simulink model "planmodel2023"  (R2023b)
settings: Solver=ode4  StartTime=0.0  StopTime=200  FixedStep=0.001  RelTol=1e-3
values from neighbouring files (symbols this model uses):
  a0 = 340.294    [plan.m]    (also in plan.mat)
  b_ref = 2.0    (= 2)    [plan.m]    (also in plan.mat)
  c_gear = [0.8e4, 1.4e4, 1.4e4]    [plan.m]    (also in plan.mat = [8000 14000 14000])
  c_lat = [1.4e4, 2.2e4, 2.2e4]    [plan.m]    (also in plan.mat = [14000 22000 22000])
  c_ref = 0.9    [plan.m]    (also in plan.mat)
  c_roll = [0.020, 0.018, 0.018]    [plan.m]    (also in plan.mat = [0.02 0.018 0.018])
  CD0 = 0.045    [plan.m]    (also in plan.mat)
  CL0 = 0.083    [plan.m]    (also in plan.mat)
  CLa = 2.50    (= 2.5)    [plan.m]    (also in plan.mat = 3.8)
  Clb = -0.08    [plan.m]    (also in plan.mat)
  Clda = 0.20    (= 0.2)    [plan.m]    (also in plan.mat = -0.2)
  CLde = 0.25    [plan.m]    (also in plan.mat = 0.28)
  Clp = -0.70    (= -0.7)    [plan.m]    (also in plan.mat)
  CLq = 3.00    (= 3)    [plan.m]    (also in plan.mat = 4.5)
  Clr = 0    [plan.m]    (also in plan.mat = 0.08)
  Cm0 = 0.112    [plan.m]    (also in plan.mat = 0.06)
  Cma = -0.8    [plan.m]    (also in plan.mat)
  Cmde = 0.90    (= 0.9)    [plan.m]    (also in plan.mat = -0.9)
  Cmq = -18.0    (= -18)    [plan.m]    (also in plan.mat)
  Cnb = -0.25    [plan.m]    (also in plan.mat = 0.25)
  Cndr = 0.15    [plan.m]    (also in plan.mat = -0.15)
  Cnp = 0    [plan.m]    (also in plan.mat = -0.04)
  Cnr = -0.45    [plan.m]    (also in plan.mat)
  CSb = -0.8    [plan.m]    (also in plan.mat = -0.7)
  CSdr = 0.18    [plan.m]    (also in plan.mat)
  CSr = 0.15    [plan.m]    (also in plan.mat = 0.12)
  D0 = 800    [plan.m]    (also in plan.mat)
  da_max = 25    [plan.m]    (also in plan.mat)
  da_min = -da_max    (= -25)    [plan.m]    (also in plan.mat)
  de_max = 25    [plan.m]    (also in plan.mat)
  de_min = -de_max    (= -25)    [plan.m]    (also in plan.mat)
  DH = pi / 180    (= 0.0174532925199)    [plan.m]    (also in plan.mat)
  dr_max = 25    [plan.m]    (also in plan.mat)
  dr_min = -dr_max    (= -25)    [plan.m]    (also in plan.mat)
  g = 9.80665    [plan.m]    (also in plan.mat)
  gamma0 = 0.0    (= 0)    [plan.m]
  ground_y = 0.0    (= 0)    [plan.m]
  HD = 180 / pi    (= 57.2957795131)    [plan.m]    (also in plan.mat)
  Ixx = 120.0    (= 120)    [plan.m]    (also in plan.mat)
  Iyy = 480.0    (= 480)    [plan.m]    (also in plan.mat)
  Izz = 520.0    (= 520)    [plan.m]    (also in plan.mat)
  K = 0.080    (= 0.08)    [plan.m]    (also in plan.mat = 0.12)
  K_alpha = 7.67884615385    [plan.mat]
  k_gear = [1.0e5, 3.0e5, 3.0e5]    [plan.m]    (also in plan.mat = [100000 300000 300000])
  k_theta0 = 0.0    (= 0)    [plan.m]
  Kb_to_wy = 10.6510416667    [plan.mat]
  Kn_pitch = 0.117046638908    [plan.mat]
  Kn_to_beta = 0.461367696223    [plan.mat]
  Kw_pitch = -0.524061476442    [plan.mat]
  Kw_to_dr = -1.30612244898    [plan.mat]
  m = 600.0    (= 600)    [plan.m]    (also in plan.mat)
  mu_brake = [0.0, 0.55, 0.55]    [plan.m]    (also in plan.mat = [0 0.55 0.55])
  omigax0 = 0    [plan.m]
  omigay0 = 0    [plan.m]
  omigaz0 = 0    [plan.m]
  psi0 = 0.3/57.3    (= 0.00523560209424)    [plan.m]    (also in plan.mat = 0)
  r_left_b = r_gear_b(:,2)    [plan.m]    (also in plan.mat = [-0.333333333333 -0.8 0.65])
  r_nose_b = r_gear_b(:,1)    [plan.m]    (also in plan.mat = [2 0 0.65])
  r_right_b = r_gear_b(:,3)    [plan.m]    (also in plan.mat = [-0.333333333333 0.8 0.65])
  rho0 = 1.225    [plan.m]    (also in plan.mat)
  S_ref = 1.2    [plan.m]    (also in plan.mat)
  v_eps = 0.20    (= 0.2)    [plan.m]    (also in plan.mat)
  V_min = 1    [plan.m]    (also in plan.mat = 3)
  V_test = 200    [plan.mat]
  Vx0_b = 0.0    (= 0)    [plan.m]
  Vy0_b = 0.0    (= 0)    [plan.m]
  Vz0_b = 0.0    (= 0)    [plan.m]
  wheel_radius = 0.18    [plan.m]    (also in plan.mat)
  WOW_on = 0.000    (= 0)    [plan.m]    (also in plan.mat)
  Xg0 = 0.0    (= 0)    [plan.m]    (also in plan.mat)
  Yg0 = ground_y + wheel_radius - r_gear_b(2,1) - static_deflection    [plan.m]    (also in plan.mat = 0)
  Zg0 = 1.0    (= 1)    [plan.m]    (also in plan.mat = -0.8215943)
libraries: matrix_library x18, slpidlib x1
(part 2 of 3)

== system planmodel2023/control/航向通道控制器/偏航通道 ==
  nzc : Inport
  nz : Inport  Port=2
  wy : Inport  Port=3
  Constant1 : Constant
  Constant3 : Constant  Value=0
  Div : Product  Inputs=/*
  Gain : Gain  Gain=-Kn_to_beta
  Gain1 : Gain  Gain=Kb_to_wy
  Gain2 : Gain  Gain=Kw_to_dr
  Gain4 : Gain  Gain=HD
  Integrator : Integrator  ExternalReset=either
  Pk : Product
  Pn : Product
  Sat : Saturate  UpperLimit=10  LowerLimit=0.25
  Saturation1 : Saturate  UpperLimit=0.2*57.3  LowerLimit=-0.2*57.3
  Scope : Scope  NumInputPorts=2
  Scope1 : Scope
  Scope12 : Scope
  Scope2 : Scope  NumInputPorts=2
  Sqr : Math  Operator=square
  Sum : Sum  Inputs=|+-
  Sum1 : Sum  Inputs=|+-
  Sum2 : Sum  Inputs=|+-
  Switch2 : Switch  Threshold=40  SaturateOnIntegerOverflow=off  InputSameDT=off
  VRef : Constant  Value=V_test
  伪攻角回路 : Subsystem
  delta_r : Outport
  wires:
  nz/1 -> Sum/2, Scope/2
  nzc/1 -> Scope/1, Sum/1
  Constant1/1 -> Switch2/1
  Constant3/1 -> Switch2/3
  [Vg] -> Div/2, Switch2/2
  Gain4/1 -> Scope12/1
  [psi_eular] -> Gain4/1
  wy/1 -> Scope2/2, Sum2/2, 伪攻角回路/1(wy)
  伪攻角回路/1(beta_c) -> Sum1/2
  Sum1/1 -> Gain1/1
  Gain1/1 -> Scope2/1, Sum2/1
  Sum2/1 -> Gain2/1
  Sum/1 -> Gain/1
  Integrator/1 -> Saturation1/1
  Saturation1/1 -> Sum1/1
  Switch2/1 -> Integrator/2
  VRef/1 -> Div/1
  Div/1 -> Sqr/1
  Sqr/1 -> Sat/1
  Sat/1 -> Pn/2, Pk/2
  Gain2/1 -> Pk/1
  Pk/1 -> delta_r/1, Scope1/1
  Gain/1 -> Pn/1
  Pn/1 -> Integrator/1

== system planmodel2023/control/航向通道控制器/地面转向控制 ==
  Z_cmd : Inport
  Gain : Gain  Gain=0.8
  Gain4 : Gain  Gain=HD
  K_z : Constant  Value=0.04
  Product : Product
  Saturation1 : Saturate  UpperLimit=5  LowerLimit=-5
  Scope : Scope  NumInputPorts=2
  Scope12 : Scope
  Scope25 : Scope
  Sum : Sum  Inputs=|+-
  Sum1 : Sum  Inputs=|++
  Transfer Fcn : TransferFcn  Denominator=[0.1 1]
  delta_s(H) : Outport
  wires:
  Z_cmd/1 -> Scope/1, Sum/1
  [Z_positon] -> Scope/2, Sum/2
  K_z/1 -> Product/1
  [delta_s] -> Scope25/1
  [psi_eular] -> Gain/1
  Gain4/1 -> Scope12/1
  [psi_eular] -> Gain4/1
  Gain/1 -> Sum1/2
  Sum/1 -> Saturation1/1
  Product/1 -> Sum1/1
  Saturation1/1 -> Product/2
  Sum1/1 -> Transfer Fcn/1
  Transfer Fcn/1 -> delta_s(H)/1

== system planmodel2023/control/航向通道控制器1/偏航通道 ==
  nzc : Inport
  nz : Inport  Port=2
  wy : Inport  Port=3
  Constant1 : Constant
  Constant3 : Constant  Value=0
  Gain : Gain  Gain=-Kn_to_beta
  Gain1 : Gain  Gain=Kb_to_wy
  Gain2 : Gain  Gain=Kw_to_dr
  Gain4 : Gain  Gain=HD
  Integrator : Integrator  ExternalReset=either
  Saturation1 : Saturate  UpperLimit=0.2*57.3  LowerLimit=-0.2*57.3
  Scope : Scope  NumInputPorts=2
  Scope1 : Scope
  Scope12 : Scope
  Scope2 : Scope  NumInputPorts=2
  Sum : Sum  Inputs=|+-
  Sum1 : Sum  Inputs=|+-
  Sum2 : Sum  Inputs=|+-
  Switch2 : Switch  Threshold=40  SaturateOnIntegerOverflow=off  InputSameDT=off
  伪攻角回路 : Subsystem
  delta_r : Outport
  wires:
  nz/1 -> Scope/2, Sum/2
  nzc/1 -> Scope/1, Sum/1
  Constant1/1 -> Switch2/1
  Constant3/1 -> Switch2/3
  [Vg] -> Switch2/2
  Gain4/1 -> Scope12/1
  [psi_eular] -> Gain4/1
  wy/1 -> Scope2/2, Sum2/2, 伪攻角回路/1(wy)
  伪攻角回路/1(beta_c) -> Sum1/2
  Sum1/1 -> Gain1/1
  Gain1/1 -> Scope2/1, Sum2/1
  Sum2/1 -> Gain2/1
  Gain2/1 -> Scope1/1, delta_r/1
  Gain/1 -> Integrator/1
  Sum/1 -> Gain/1
  Integrator/1 -> Saturation1/1
  Saturation1/1 -> Sum1/1
  Switch2/1 -> Integrator/2

== system planmodel2023/control/航向通道控制器1/地面转向控制 ==
  Z_cmd : Inport
  Gain : Gain  Gain=0.8
  Gain4 : Gain  Gain=HD
  K_z : Constant  Value=0.04
  Product : Product
  Saturation1 : Saturate  UpperLimit=5  LowerLimit=-5
  Scope : Scope  NumInputPorts=2
  Scope12 : Scope
  Scope25 : Scope
  Sum : Sum  Inputs=|+-
  Sum1 : Sum  Inputs=|++
  delta_s(H) : Outport
  wires:
  Z_cmd/1 -> Scope/1, Sum/1
  [Z_positon] -> Scope/2, Sum/2
  K_z/1 -> Product/1
  [delta_s] -> Scope25/1
  [psi_eular] -> Gain/1
  Gain4/1 -> Scope12/1
  [psi_eular] -> Gain4/1
  Gain/1 -> Sum1/2
  Sum/1 -> Saturation1/1
  Product/1 -> Sum1/1
  Saturation1/1 -> Product/2
  Sum1/1 -> delta_s(H)/1

== system planmodel2023/6DOF-MODEL/AERO-PARAMETER/无量纲化角速率/Subsystem ==
  wy1 : Inport
  Va : Inport  Port=2
  Constant4 : Constant  Value=b_ref
  Divide : Product  Inputs=*/
  Gain : Gain  Gain=2
  Product : Product
  r_hat : Outport
  wires:
  Va/1 -> Gain/1
  wy1/1 -> Product/1
  Constant4/1 -> Product/2
  Product/1 -> Divide/1
  Divide/1 -> r_hat/1
  Gain/1 -> Divide/2

== system planmodel2023/6DOF-MODEL/AERO-PARAMETER/无量纲化角速率/Subsystem1 ==
  wz1 : Inport
  Va : Inport  Port=2
  Constant4 : Constant  Value=c_ref
  Divide : Product  Inputs=*/
  Gain : Gain  Gain=2
  Product : Product
  Scope : Scope
  q_hat : Outport
  wires:
  Va/1 -> Gain/1
  wz1/1 -> Scope/1, Product/1
  Constant4/1 -> Product/2
  Product/1 -> Divide/1
  Divide/1 -> q_hat/1
  Gain/1 -> Divide/2

== system planmodel2023/6DOF-MODEL/AERO-PARAMETER/无量纲化角速率/Subsystem2 ==
  wx1 : Inport
  Va : Inport  Port=2
  Constant4 : Constant  Value=b_ref
  Divide : Product  Inputs=*/
  Gain : Gain  Gain=2
  Product : Product
  p_hat : Outport
  wires:
  Va/1 -> Gain/1
  wx1/1 -> Product/1
  Constant4/1 -> Product/2
  Product/1 -> Divide/1
  Divide/1 -> p_hat/1
  Gain/1 -> Divide/2

== system planmodel2023/6DOF-MODEL/动力学/v在体系下的分量/Subsystem ==
  Fx/m : Inport
  wy1 : Inport  Port=2
  wz1 : Inport  Port=3
  vz : Inport  Port=4
  vy : Inport  Port=5
  Product1 : Product
  Product4 : Product
  Subtract1 : Sum  Inputs=+-
  Subtract3 : Sum  Inputs=+-
  vx_dot : Outport
  wires:
  Fx/m/1 -> Subtract3/1
  Subtract3/1 -> vx_dot/1
  Subtract1/1 -> Subtract3/2
  vy/1 -> Product4/2
  wz1/1 -> Product4/1
  Product4/1 -> Subtract1/2
  wy1/1 -> Product1/1
  vz/1 -> Product1/2
  Product1/1 -> Subtract1/1

== system planmodel2023/6DOF-MODEL/动力学/v在体系下的分量/Subsystem1 ==
  Fy/m : Inport
  wx1 : Inport  Port=2
  wz1 : Inport  Port=3
  vx : Inport  Port=4
  vz : Inport  Port=5
  Product1 : Product
  Product4 : Product
  Subtract2 : Sum  Inputs=+-
  Subtract3 : Sum  Inputs=+-
  vy_dot : Outport
  wires:
  Fy/m/1 -> Subtract3/1
  Subtract3/1 -> vy_dot/1
  vx/1 -> Product4/1
  wz1/1 -> Product4/2
  wx1/1 -> Product1/1
  vz/1 -> Product1/2
  Product4/1 -> Subtract2/1
  Product1/1 -> Subtract2/2
  Subtract2/1 -> Subtract3/2

== system planmodel2023/6DOF-MODEL/动力学/v在体系下的分量/Subsystem2 ==
  Fz/m : Inport
  wx1 : Inport  Port=2
  wy1 : Inport  Port=3
  vx : Inport  Port=4
  vy : Inport  Port=5
  Product1 : Product
  Product2 : Product
  Subtract2 : Sum  Inputs=+-
  Subtract3 : Sum  Inputs=+-
  vz_dot : Outport
  wires:
  Fz/m/1 -> Subtract3/1
  Subtract3/1 -> vz_dot/1
  Subtract2/1 -> Subtract3/2
  Product1/1 -> Subtract2/1
  wx1/1 -> Product1/1
  vy/1 -> Product1/2
  wy1/1 -> Product2/1
  vx/1 -> Product2/2
  Product2/1 -> Subtract2/2

== system planmodel2023/6DOF-MODEL/动力学/体系旋转角速度/Subsystem ==
  MX : Inport
  wz1 : Inport  Port=2
  wy1 : Inport  Port=3
  Constant : Constant  Value=Ixx
  Constant1 : Constant  Value=Izz
  Constant2 : Constant  Value=Iyy
  Divide : Product  Inputs=*/
  Integrator : Integrator  InitialCondition=omigax0
  Product : Product
  Product1 : Product
  Subtract : Sum  Inputs=+-
  Sum : Sum  Inputs=|+-
  wx1 : Outport
  wires:
  MX/1 -> Sum/1
  Sum/1 -> Divide/1
  Constant/1 -> Divide/2
  Subtract/1 -> Product/1
  wz1/1 -> Product1/1
  wy1/1 -> Product1/2
  Product1/1 -> Product/2
  Constant1/1 -> Subtract/1
  Constant2/1 -> Subtract/2
  Product/1 -> Sum/2
  Divide/1 -> Integrator/1
  Integrator/1 -> wx1/1

== system planmodel2023/6DOF-MODEL/动力学/体系旋转角速度/Subsystem1 ==
  MY : Inport
  wx1 : Inport  Port=2
  wz1 : Inport  Port=3
  Constant : Constant  Value=Iyy
  Constant1 : Constant  Value=Ixx
  Constant2 : Constant  Value=Izz
  Divide : Product  Inputs=*/
  Integrator : Integrator  InitialCondition=omigay0
  Product : Product
  Product1 : Product
  Subtract : Sum  Inputs=+-
  Sum : Sum  Inputs=|+-
  wy1 : Outport
  wires:
  MY/1 -> Sum/1
  Sum/1 -> Divide/1
  Constant/1 -> Divide/2
  Subtract/1 -> Product/1
  wx1/1 -> Product1/1
  wz1/1 -> Product1/2
  Product1/1 -> Product/2
  Constant1/1 -> Subtract/1
  Constant2/1 -> Subtract/2
  Product/1 -> Sum/2
  Divide/1 -> Integrator/1
  Integrator/1 -> wy1/1

== system planmodel2023/6DOF-MODEL/动力学/体系旋转角速度/Subsystem2 ==
  MZ : Inport
  wx1 : Inport  Port=2
  wy1 : Inport  Port=3
  Constant : Constant  Value=Izz
  Constant1 : Constant  Value=Iyy
  Constant2 : Constant  Value=Ixx
  Divide : Product  Inputs=*/
  Integrator : Integrator  InitialCondition=omigaz0
  Product : Product
  Product1 : Product
  Subtract : Sum  Inputs=+-
  Sum : Sum  Inputs=|+-
  wz1 : Outport
  wires:
  MZ/1 -> Sum/1
  Sum/1 -> Divide/1
  Constant/1 -> Divide/2
  Subtract/1 -> Product/1
  wx1/1 -> Product1/1
  wy1/1 -> Product1/2
  Product1/1 -> Product/2
  Constant1/1 -> Subtract/1
  Constant2/1 -> Subtract/2
  Product/1 -> Sum/2
  Divide/1 -> Integrator/1
  Integrator/1 -> wz1/1

== system planmodel2023/6DOF-MODEL/动力学/姿态角/Subsystem ==
  wx1 : Inport
  wy1 : Inport  Port=2
  wz1 : Inport  Port=3
  Integrator : Integrator  InitialCondition=gamma0
  Product : Product
  Product1 : Product
  Product2 : Product
  Subtract : Sum  Inputs=+-
  Sum : Sum  Inputs=|+-
  Trigonometric Function1 : Trigonometry  Operator=cos
  Trigonometric Function2 : Trigonometry
  Trigonometric Function8 : Trigonometry  Operator=tan
  gamma(eular) : Outport
  wires:
  wx1/1 -> Sum/1
  [gamma_eular] -> Trigonometric Function2/1, Trigonometric Function1/1
  Trigonometric Function1/1 -> Product/2
  wy1/1 -> Product/1
  Trigonometric Function2/1 -> Product1/1
  wz1/1 -> Product1/2
  Product/1 -> Subtract/1
  Product1/1 -> Subtract/2
  Subtract/1 -> Product2/2
  [theta_eular] -> Trigonometric Function8/1
  Trigonometric Function8/1 -> Product2/1
  Sum/1 -> Integrator/1
  Integrator/1 -> gamma(eular)/1
  Product2/1 -> Sum/2

== system planmodel2023/6DOF-MODEL/动力学/姿态角/Subsystem1 ==
  wy1 : Inport
  wz1 : Inport  Port=2
  Integrator : Integrator  InitialCondition=k_theta0
  Product : Product
  Product1 : Product
  Subtract : Sum
  Trigonometric Function1 : Trigonometry
  Trigonometric Function2 : Trigonometry  Operator=cos
  theta(eular) : Outport
  wires:
  [gamma_eular] -> Trigonometric Function2/1, Trigonometric Function1/1
  Trigonometric Function1/1 -> Product/2
  wy1/1 -> Product/1
  Trigonometric Function2/1 -> Product1/1
  wz1/1 -> Product1/2
  Product/1 -> Subtract/1
  Product1/1 -> Subtract/2
  Subtract/1 -> Integrator/1
  Integrator/1 -> theta(eular)/1

== system planmodel2023/6DOF-MODEL/动力学/姿态角/Subsystem2 ==
  wy1 : Inport
  wz1 : Inport  Port=2
  Divide : Product  Inputs=*/
  Integrator : Integrator  InitialCondition=psi0
  Product : Product
  Product1 : Product
  Subtract : Sum  Inputs=+-
  Trigonometric Function1 : Trigonometry  Operator=cos
  Trigonometric Function2 : Trigonometry
  Trigonometric Function8 : Trigonometry  Operator=cos
  psi(eular) : Outport
  wires:
  [gamma_eular] -> Trigonometric Function2/1, Trigonometric Function1/1
  Trigonometric Function1/1 -> Product/2
  wy1/1 -> Product/1
  Trigonometric Function2/1 -> Product1/1
  wz1/1 -> Product1/2
  Product/1 -> Subtract/1
  Product1/1 -> Subtract/2
  [theta_eular] -> Trigonometric Function8/1
  Integrator/1 -> psi(eular)/1
  Subtract/1 -> Divide/1
  Trigonometric Function8/1 -> Divide/2
  Divide/1 -> Integrator/1

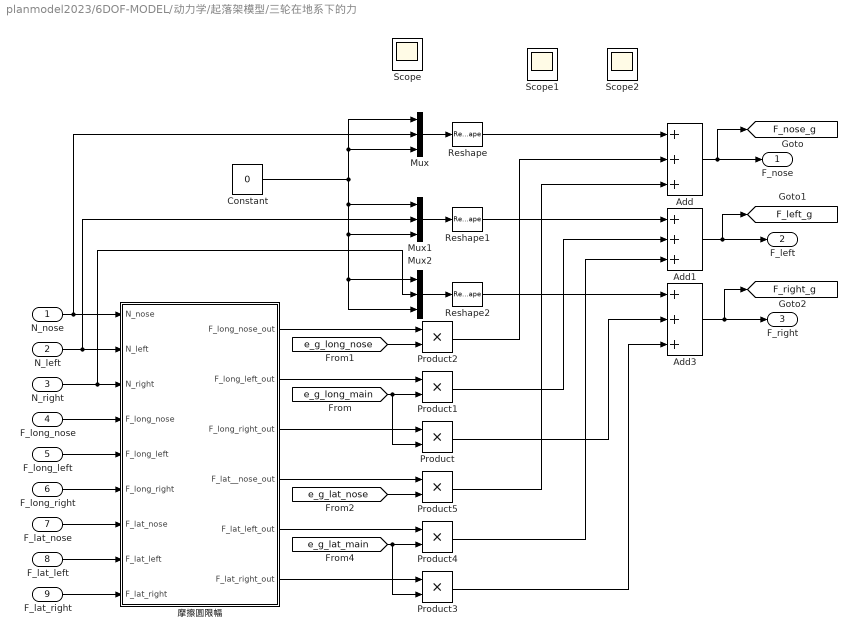
== system planmodel2023/6DOF-MODEL/动力学/起落架模型/三轮在地系下的力 ==
  N_nose : Inport
  N_left : Inport  Port=2
  N_right : Inport  Port=3
  F_long_nose : Inport  Port=4
  F_long_left : Inport  Port=5
  F_long_right : Inport  Port=6
  F_lat_nose : Inport  Port=7
  F_lat_left : Inport  Port=8
  F_lat_right : Inport  Port=9
  Add : Sum  Inputs=+++
  Add1 : Sum  Inputs=+++
  Add3 : Sum  Inputs=+++
  Constant : Constant  Value=0
  Mux : Mux  Inputs=3
  Mux1 : Mux  Inputs=3
  Mux2 : Mux  Inputs=3
  Product{,1..5} (6 alike) : Product
  Reshape : Reshape  OutputDimensionality=Column vector (2-D)
  Reshape1 : Reshape  OutputDimensionality=Column vector (2-D)
  Reshape2 : Reshape  OutputDimensionality=Column vector (2-D)
  Scope : Scope
  Scope1 : Scope
  Scope2 : Scope
  摩擦圆限幅 : Subsystem
  F_nose : Outport
  F_left : Outport  Port=2
  F_right : Outport  Port=3
  tag scope: F_left_g=global, F_nose_g=global, F_right_g=global
  wires:
  Product1/1 -> Add1/2
  Constant/1 -> Mux2/3, Mux2/1, Mux1/3, Mux1/1, Mux/1, Mux/3
  [e_g_long_nose] -> Product2/2
  [e_g_long_main] -> Product/2, Product1/2
  Product5/1 -> Add/3
  Product2/1 -> Add/2
  Product/1 -> Add3/2
  [e_g_lat_nose] -> Product5/2
  [e_g_lat_main] -> Product3/2, Product4/2
  Product4/1 -> Add1/3
  Product3/1 -> Add3/3
  Add/1 -> [F_nose_g], F_nose/1
  Add1/1 -> [F_left_g], F_left/1
  Add3/1 -> [F_right_g], F_right/1
  Mux/1 -> Reshape/1
  Mux2/1 -> Reshape2/1
  Reshape2/1 -> Add3/1
  Reshape1/1 -> Add1/1
  Mux1/1 -> Reshape1/1
  Reshape/1 -> Add/1
  N_nose/1 -> Mux/2, 摩擦圆限幅/1(N_nose)
  N_left/1 -> Mux1/2, 摩擦圆限幅/2(N_left)
  N_right/1 -> Mux2/2, 摩擦圆限幅/3(N_right)
  F_long_nose/1 -> 摩擦圆限幅/4(F_long_nose)
  F_long_left/1 -> 摩擦圆限幅/5(F_long_left)
  F_long_right/1 -> 摩擦圆限幅/6(F_long_right)
  F_lat_nose/1 -> 摩擦圆限幅/7(F_lat_nose)
  F_lat_left/1 -> 摩擦圆限幅/8(F_lat_left)
  F_lat_right/1 -> 摩擦圆限幅/9(F_lat_right)
  摩擦圆限幅/1(F_long_nose_out) -> Product2/1
  摩擦圆限幅/4(F_lat__nose_out) -> Product5/1
  摩擦圆限幅/2(F_long_left_out) -> Product1/1
  摩擦圆限幅/5(F_lat_left_out) -> Product4/1
  摩擦圆限幅/3(F_long_right_out) -> Product/1
  摩擦圆限幅/6(F_lat_right_out) -> Product3/1

== system planmodel2023/6DOF-MODEL/动力学/起落架模型/三轮接地判定 ==
  Logical Operator : Logic  AllPortsSameDT=off  OutDataTypeStr=boolean
  Logical Operator1 : Logic  Operator=NOR  Inputs=3  AllPortsSameDT=off  OutDataTypeStr=boolean
  tag scope: contact_main=global, no_contact=global
  wires:
  Logical Operator/1 -> [contact_main]
  [contact_nose] -> Logical Operator1/1
  [contact_left] -> Logical Operator1/2, Logical Operator/1
  [contact_right] -> Logical Operator1/3, Logical Operator/2
  Logical Operator1/1 -> [no_contact]

== system planmodel2023/6DOF-MODEL/动力学/起落架模型/侧向力 ==
  delt-s(H) : Inport
  Constant : Constant  Value=c_lat
  Demux : Demux  Outputs=3
  Gain : Gain  Gain=-1
  Gain1 : Gain  Gain=-1
  Gain2 : Gain  Gain=-1
  Product : Product
  Product1 : Product
  Product2 : Product
  Subsystem : Subsystem
  Subsystem1 : Subsystem
  Subsystem2 : Subsystem
  Subsystem3 : Subsystem
  F_lat_nose : Outport
  F_lat_left : Outport  Port=2
  F_lat_right : Outport  Port=3
  wires:
  delt-s(H)/1 -> Subsystem/1(delt-s(H))
  Constant/1 -> Demux/1
  Subsystem/1(V_lat_nose) -> Product/1
  Demux/1 -> Product/2
  Subsystem/2(V_lat_left) -> Product1/1
  Subsystem/3(V_lat_right) -> Product2/1
  Demux/2 -> Product1/2
  Demux/3 -> Product2/2
  Product/1 -> Gain/1
  Product1/1 -> Gain1/1
  Product2/1 -> Gain2/1
  Gain/1 -> Subsystem2/1(In1)
  Subsystem2/1(F_lat_nose) -> F_lat_nose/1
  Gain1/1 -> Subsystem1/1(In1)
  Subsystem1/1(F_lat_left) -> F_lat_left/1
  Gain2/1 -> Subsystem3/1(In1)
  Subsystem3/1(F_lat_right) -> F_lat_right/1

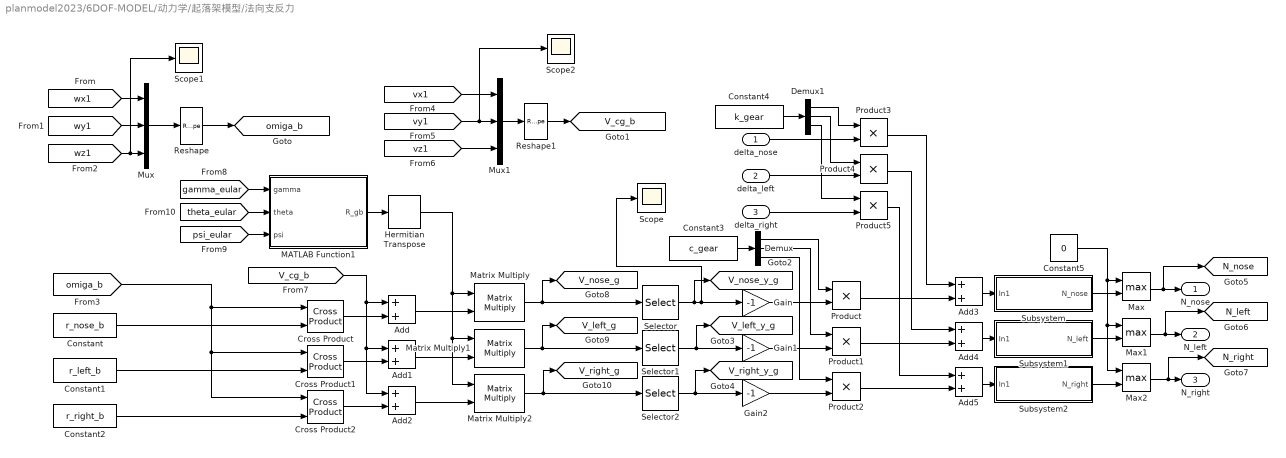
== system planmodel2023/6DOF-MODEL/动力学/起落架模型/法向支反力 ==
  delta_nose : Inport
  delta_left : Inport  Port=2
  delta_right : Inport  Port=3
  Add{,1..5} (6 alike) : Sum
  Constant : Constant  Value=r_nose_b
  Constant1 : Constant  Value=r_left_b
  Constant2 : Constant  Value=r_right_b
  Constant3 : Constant  Value=c_gear
  Constant4 : Constant  Value=k_gear
  Constant5 : Constant  Value=0
  Cross Product : matrix_library/Cross Product
  Cross Product1 : matrix_library/Cross Product
  Cross Product2 : matrix_library/Cross Product
  Demux : Demux  Outputs=3
  Demux1 : Demux  Outputs=3
  Gain : Gain  Gain=-1
  Gain1 : Gain  Gain=-1
  Gain2 : Gain  Gain=-1
  Hermitian Transpose : matrix_library/Hermitian Transpose
  MATLAB Function1 : MATLAB Function  TreatAsAtomicUnit=on
  Matrix Multiply : Product  Multiplication=Matrix(*)
  Matrix Multiply1 : Product  Multiplication=Matrix(*)
  Matrix Multiply2 : Product  Multiplication=Matrix(*)
  Max : MinMax  Function=max  Inputs=2
  Max1 : MinMax  Function=max  Inputs=2
  Max2 : MinMax  Function=max  Inputs=2
  Mux : Mux  Inputs=3
  Mux1 : Mux  Inputs=3
  Product{,1..5} (6 alike) : Product
  Reshape : Reshape  OutputDimensionality=Column vector (2-D)
  Reshape1 : Reshape  OutputDimensionality=Column vector (2-D)
  Scope : Scope
  Scope1 : Scope
  Scope2 : Scope
  Selector : Selector  InputPortWidth=3  IndexOptions=Index vector (dialog)  Indices=2  OutputSizes=1
  Selector1 : Selector  InputPortWidth=3  IndexOptions=Index vector (dialog)  Indices=2  OutputSizes=1
  Selector2 : Selector  InputPortWidth=3  IndexOptions=Index vector (dialog)  Indices=2  OutputSizes=1
  Subsystem : Subsystem
  Subsystem1 : Subsystem
  Subsystem2 : Subsystem
  N_nose : Outport
  N_left : Outport  Port=2
  N_right : Outport  Port=3
  tag scope: N_left=global, N_nose=global, N_right=global, V_cg_b=global, V_left_g=global, V_left_y_g=global, V_nose_g=global, V_nose_y_g=global, V_right_g=global, V_right_y_g=global, omiga_b=global
  wires:
  [wx1] -> Mux/1
  [wz1] -> Scope1/1, Mux/3
  [wy1] -> Mux/2
  Mux/1 -> Reshape/1
  Reshape/1 -> [omiga_b]
  Constant2/1 -> Cross Product2/2
  Constant1/1 -> Cross Product1/2
  Constant/1 -> Cross Product/2
  [omiga_b] -> Cross Product1/1, Cross Product2/1, Cross Product/1
  [vy1] -> Scope2/1, Mux1/2
  [vx1] -> Mux1/1
  [vz1] -> Mux1/3
  Mux1/1 -> Reshape1/1
  Reshape1/1 -> [V_cg_b]
  Cross Product/1 -> Add/2
  Cross Product1/1 -> Add1/2
  Cross Product2/1 -> Add2/2
  [V_cg_b] -> Add/1, Add1/1, Add2/1
  MATLAB Function1/1(R_gb) -> Hermitian Transpose/1
  [gamma_eular] -> MATLAB Function1/1(gamma)
  Add1/1 -> Matrix Multiply1/2
  Add2/1 -> Matrix Multiply2/2
  Add/1 -> Matrix Multiply/2
  Hermitian Transpose/1 -> Matrix Multiply/1, Matrix Multiply1/1, Matrix Multiply2/1
  Matrix Multiply/1 -> [V_nose_g], Selector/1
  Matrix Multiply1/1 -> [V_left_g], Selector1/1
  Matrix Multiply2/1 -> [V_right_g], Selector2/1
  Selector2/1 -> Gain2/1, [V_right_y_g]
  Selector1/1 -> Gain1/1, [V_left_y_g]
  Selector/1 -> Scope/1, Gain/1, [V_nose_y_g]
  Product/1 -> Add3/2
  Product3/1 -> Add3/1
  Product1/1 -> Add4/2
  Product2/1 -> Add5/2
  Product4/1 -> Add4/1
  Product5/1 -> Add5/1
  Add4/1 -> Subsystem1/1(In1)
  Add5/1 -> Subsystem2/1(In1)
  delta_nose/1 -> Product3/2
  delta_left/1 -> Product4/2
  delta_right/1 -> Product5/2
  Gain/1 -> Product/2
  Gain1/1 -> Product1/2
  Gain2/1 -> Product2/2
  [theta_eular] -> MATLAB Function1/2(theta)
  [psi_eular] -> MATLAB Function1/3(psi)
  Constant3/1 -> Demux/1
  Demux/1 -> Product/1
  Demux/3 -> Product2/1
  Constant4/1 -> Demux1/1
  Demux1/1 -> Product3/1
  Demux1/2 -> Product4/1
  Demux1/3 -> Product5/1
  Add3/1 -> Subsystem/1(In1)
  Max/1 -> [N_nose], N_nose/1
  Subsystem1/1(N_left) -> Max1/2
  Max1/1 -> [N_left], N_left/1
  Subsystem/1(N_nose) -> Max/2
  Subsystem2/1(N_right) -> Max2/2
  Max2/1 -> [N_right], N_right/1
  Constant5/1 -> Max2/1, Max1/1, Max/1
  Demux/2 -> Product1/1

== system planmodel2023/6DOF-MODEL/动力学/起落架模型/纵向力 ==
  delta_s(H) : Inport
  u_brake : Inport  Port=2
  Subsystem : Subsystem
  Subsystem1 : Subsystem
  F_long_nose : Outport
  F_long_left : Outport  Port=2
  F_long_right : Outport  Port=3
  wires:
  delta_s(H)/1 -> Subsystem/1(delt-s(H))
  Subsystem/1(V_long_nose) -> Subsystem1/1(V_long_nose)
  Subsystem/2(V_long_left) -> Subsystem1/2(V_long_left)
  Subsystem/3(V_long_right) -> Subsystem1/3(V_long_right)
  u_brake/1 -> Subsystem1/4(u_brake)
  Subsystem1/1(F_long_nose) -> F_long_nose/1
  Subsystem1/2(F_long_left) -> F_long_left/1
  Subsystem1/3(F_long_right) -> F_long_right/1

== system planmodel2023/6DOF-MODEL/动力学/起落架模型/起落架三轮质心在地系下位置 ==
  Add : Sum
  Add1 : Sum
  Add2 : Sum
  Constant : Constant  Value=r_nose_b
  Constant1 : Constant  Value=r_left_b
  Constant2 : Constant  Value=r_right_b
  MATLAB Function1 : MATLAB Function  TreatAsAtomicUnit=on
  Matrix Multiply : Product  Multiplication=Matrix(*)
  Matrix Multiply1 : Product  Multiplication=Matrix(*)
  Matrix Multiply2 : Product  Multiplication=Matrix(*)
  Mux : Mux  Inputs=3
  Scope : Scope
  Scope1 : Scope
  Scope2 : Scope
  Selector : Selector  InputPortWidth=3  IndexOptions=Index vector (dialog)  Indices=2  OutputSizes=1
  Transpose : matrix_library/Transpose
  Nose_pos_g : Outport
  Left_pos_g : Outport  Port=2
  Right_pos_g : Outport  Port=3
  tag scope: Left_pos_g=global, Nose_position_g=global, Right_pos_g=global
  wires:
  Constant1/1 -> Matrix Multiply1/2
  Transpose/1 -> Matrix Multiply2/1, Matrix Multiply1/1, Matrix Multiply/1
  [psi_eular] -> MATLAB Function1/3(psi)
  [gamma_eular] -> Scope2/1, MATLAB Function1/1(gamma)
  Constant2/1 -> Matrix Multiply2/2
  Matrix Multiply1/1 -> Add1/2
  Constant/1 -> Matrix Multiply/2
  [theta_eular] -> MATLAB Function1/2(theta)
  MATLAB Function1/1(R_gb) -> Transpose/1
  Matrix Multiply/1 -> Add/2
  Matrix Multiply2/1 -> Add2/2
  [Z_positon] -> Mux/3
  [Y_positon] -> Scope1/1, Mux/2
  [X_positon] -> Mux/1
  Mux/1 -> Add/1, Add1/1, Add2/1
  Add/1 -> Selector/1, Nose_pos_g/1, [Nose_position_g]
  Add1/1 -> Left_pos_g/1, [Left_pos_g]
  Add2/1 -> Right_pos_g/1, [Right_pos_g]
  Selector/1 -> Scope/1

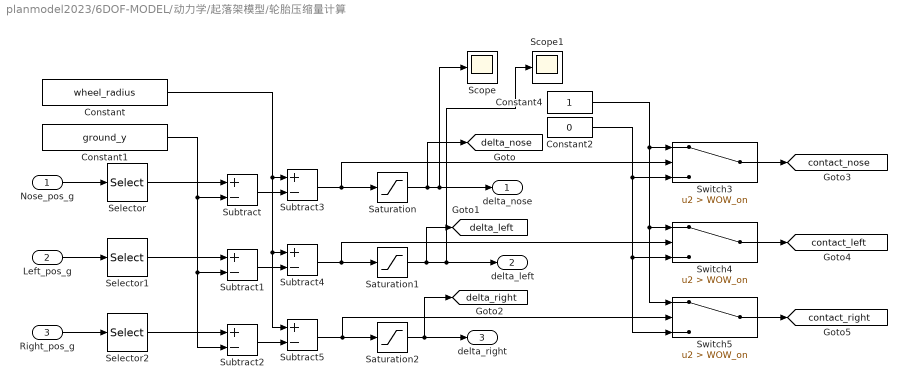
== system planmodel2023/6DOF-MODEL/动力学/起落架模型/轮胎压缩量计算 ==
  Nose_pos_g : Inport
  Left_pos_g : Inport  Port=2
  Right_pos_g : Inport  Port=3
  Constant : Constant  Value=wheel_radius
  Constant1 : Constant  Value=ground_y
  Constant2 : Constant  Value=0
  Constant4 : Constant
  Saturation : Saturate  UpperLimit=wheel_radius  LowerLimit=0
  Saturation1 : Saturate  UpperLimit=wheel_radius  LowerLimit=0
  Saturation2 : Saturate  UpperLimit=wheel_radius  LowerLimit=0
  Scope : Scope
  Scope1 : Scope
  Selector : Selector  InputPortWidth=3  IndexOptions=Index vector (dialog)  Indices=2  OutputSizes=1
  Selector1 : Selector  InputPortWidth=3  IndexOptions=Index vector (dialog)  Indices=2  OutputSizes=1
  Selector2 : Selector  InputPortWidth=3  IndexOptions=Index vector (dialog)  Indices=2  OutputSizes=1
  Subtract{,1..5} (6 alike) : Sum  Inputs=+-
  Switch3 : Switch  Criteria=u2 > Threshold  Threshold=WOW_on  SaturateOnIntegerOverflow=off  InputSameDT=off
  Switch4 : Switch  Criteria=u2 > Threshold  Threshold=WOW_on  SaturateOnIntegerOverflow=off  InputSameDT=off
  Switch5 : Switch  Criteria=u2 > Threshold  Threshold=WOW_on  SaturateOnIntegerOverflow=off  InputSameDT=off
  delta_nose : Outport
  delta_left : Outport  Port=2
  delta_right : Outport  Port=3
  tag scope: contact_left=global, contact_nose=global, contact_right=global, delta_left=global, delta_nose=global, delta_right=global
  wires:
  Nose_pos_g/1 -> Selector/1
  Left_pos_g/1 -> Selector1/1
  Right_pos_g/1 -> Selector2/1
  Selector/1 -> Subtract/1
  Selector1/1 -> Subtract1/1
  Selector2/1 -> Subtract2/1
  Constant1/1 -> Subtract/2, Subtract1/2, Subtract2/2
  Subtract/1 -> Subtract3/2
  Subtract1/1 -> Subtract4/2
  Subtract2/1 -> Subtract5/2
  Constant/1 -> Subtract5/1, Subtract4/1, Subtract3/1
  Saturation/1 -> Scope/1, delta_nose/1, [delta_nose]
  Saturation1/1 -> [delta_left], delta_left/1, Scope1/1
  Saturation2/1 -> [delta_right], delta_right/1
  Subtract3/1 -> Switch3/2, Saturation/1
  Subtract4/1 -> Switch4/2, Saturation1/1
  Subtract5/1 -> Switch5/2, Saturation2/1
  Constant2/1 -> Switch3/3, Switch5/3, Switch4/3
  Constant4/1 -> Switch5/1, Switch4/1, Switch3/1
  Switch3/1 -> [contact_nose]
  Switch5/1 -> [contact_right]
  Switch4/1 -> [contact_left]

== system planmodel2023/control/俯仰通道控制器/俯仰通道/伪攻角回路 ==
  wz : Inport
  Constant : Constant
  Integrator : Integrator  ExternalReset=either
  Product : Product
  Subsystem : Subsystem
  Sum : Sum  Inputs=|+-
  Sum3 : Sum  Inputs=|+-
  To Workspace : ToWorkspace  VariableName=a34  SaveFormat=Timeseries  SampleTime=-1
  alpha_c : Outport
  wires:
  wz/1 -> Sum/1
  Sum/1 -> Integrator/1
  Integrator/1 -> alpha_c/1, Product/2
  Product/1 -> Sum/2
  Subsystem/1(a34) -> Product/1, To Workspace/1
  Sum3/1 -> Integrator/2
  [no_contact] -> Sum3/2
  Constant/1 -> Sum3/1

== system planmodel2023/control/航向通道控制器/偏航通道/伪攻角回路 ==
  wy : Inport
  Constant1 : Constant
  Constant3 : Constant  Value=0
  Integrator : Integrator  ExternalReset=either
  Product : Product
  Subsystem : Subsystem
  Sum : Sum  Inputs=|+-
  Switch2 : Switch  Threshold=40  SaturateOnIntegerOverflow=off  InputSameDT=off
  beta_c : Outport
  wires:
  wy/1 -> Sum/1
  Sum/1 -> Integrator/1
  Integrator/1 -> beta_c/1, Product/2
  Product/1 -> Sum/2
  Subsystem/1(b) -> Product/1
  [Vg] -> Switch2/2
  Constant1/1 -> Switch2/1
  Constant3/1 -> Switch2/3
  Switch2/1 -> Integrator/2

== system planmodel2023/control/航向通道控制器1/偏航通道/伪攻角回路 ==
  wy : Inport
  Constant1 : Constant
  Constant3 : Constant  Value=0
  Integrator : Integrator  ExternalReset=either
  Product : Product
  Subsystem : Subsystem
  Sum : Sum  Inputs=|+-
  Switch2 : Switch  Threshold=40  SaturateOnIntegerOverflow=off  InputSameDT=off
  beta_c : Outport
  wires:
  wy/1 -> Sum/1
  Sum/1 -> Integrator/1
  Integrator/1 -> beta_c/1, Product/2
  Product/1 -> Sum/2
  Subsystem/1(b) -> Product/1
  [Vg] -> Switch2/2
  Constant1/1 -> Switch2/1
  Constant3/1 -> Switch2/3
  Switch2/1 -> Integrator/2

== system planmodel2023/6DOF-MODEL/动力学/起落架模型/三轮在地系下的力/摩擦圆限幅 ==
  N_nose : Inport
  N_left : Inport  Port=2
  N_right : Inport  Port=3
  F_long_nose : Inport  Port=4
  F_long_left : Inport  Port=5
  F_long_right : Inport  Port=6
  F_lat_nose : Inport  Port=7
  F_lat_left : Inport  Port=8
  F_lat_right : Inport  Port=9
  主轮摩擦圆限幅右 : MATLAB Function  TreatAsAtomicUnit=on
  主轮摩擦圆限幅左 : MATLAB Function  TreatAsAtomicUnit=on
  前轮摩擦圆限幅 : MATLAB Function  TreatAsAtomicUnit=on
  F_long_nose_out : Outport
  F_long_left_out : Outport  Port=2
  F_long_right_out : Outport  Port=3
  F_lat__nose_out : Outport  Port=4
  F_lat_left_out : Outport  Port=5
  F_lat_right_out : Outport  Port=6
  wires:
  前轮摩擦圆限幅/1(F_long_out) -> F_long_nose_out/1
  前轮摩擦圆限幅/2(F_lat_out) -> F_lat__nose_out/1
  主轮摩擦圆限幅左/2(F_lat_out) -> F_lat_left_out/1
  主轮摩擦圆限幅左/1(F_long_out) -> F_long_left_out/1
  主轮摩擦圆限幅右/2(F_lat_out) -> F_lat_right_out/1
  主轮摩擦圆限幅右/1(F_long_out) -> F_long_right_out/1
  N_nose/1 -> 前轮摩擦圆限幅/1(N)
  F_long_nose/1 -> 前轮摩擦圆限幅/2(F_long)
  F_lat_nose/1 -> 前轮摩擦圆限幅/3(F_lat)
  F_long_left/1 -> 主轮摩擦圆限幅左/2(F_long)
  N_left/1 -> 主轮摩擦圆限幅左/1(N)
  F_lat_right/1 -> 主轮摩擦圆限幅右/3(F_lat)
  F_lat_left/1 -> 主轮摩擦圆限幅左/3(F_lat)
  F_long_right/1 -> 主轮摩擦圆限幅右/2(F_long)
  N_right/1 -> 主轮摩擦圆限幅右/1(N)

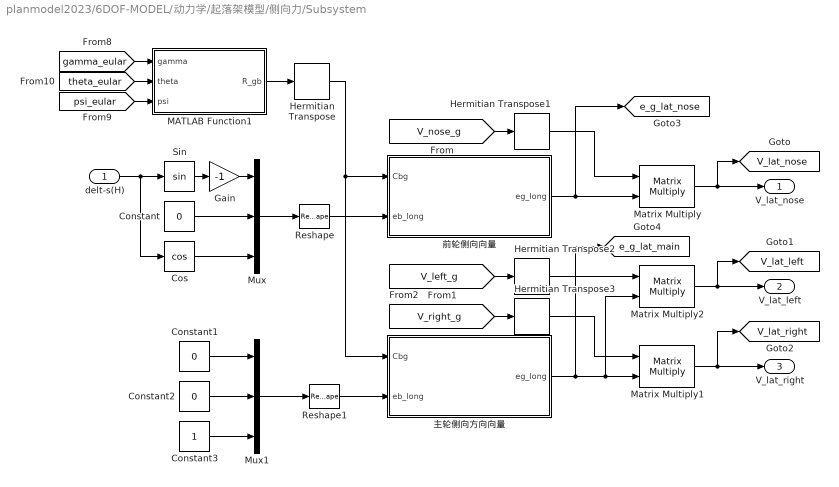
== system planmodel2023/6DOF-MODEL/动力学/起落架模型/侧向力/Subsystem ==
  delt-s(H) : Inport
  Constant : Constant  Value=0
  Constant1 : Constant  Value=0
  Constant2 : Constant  Value=0
  Constant3 : Constant
  Cos : Trigonometry  Operator=cos
  Gain : Gain  Gain=-1
  Hermitian Transpose{,1..3} (4 alike) : matrix_library/Hermitian Transpose
  MATLAB Function1 : MATLAB Function  TreatAsAtomicUnit=on
  Matrix Multiply : Product  Multiplication=Matrix(*)
  Matrix Multiply1 : Product  Multiplication=Matrix(*)
  Matrix Multiply2 : Product  Multiplication=Matrix(*)
  Mux : Mux  Inputs=3
  Mux1 : Mux  Inputs=3
  Reshape : Reshape  OutputDimensionality=Column vector (2-D)
  Reshape1 : Reshape  OutputDimensionality=Column vector (2-D)
  Sin : Trigonometry
  主轮侧向方向向量 : MATLAB Function  TreatAsAtomicUnit=on
  前轮侧向向量 : MATLAB Function  TreatAsAtomicUnit=on
  V_lat_nose : Outport
  V_lat_left : Outport  Port=2
  V_lat_right : Outport  Port=3
  tag scope: V_lat_left=global, V_lat_nose=global, V_lat_right=global, e_g_lat_main=global, e_g_lat_nose=global
  wires:
  MATLAB Function1/1(R_gb) -> Hermitian Transpose/1
  [gamma_eular] -> MATLAB Function1/1(gamma)
  Hermitian Transpose/1 -> 主轮侧向方向向量/1(Cbg), 前轮侧向向量/1(Cbg)
  Constant/1 -> Mux/2
  Mux/1 -> Reshape/1
  Constant1/1 -> Mux1/1
  Constant2/1 -> Mux1/2
  Constant3/1 -> Mux1/3
  Mux1/1 -> Reshape1/1
  [V_nose_g] -> Hermitian Transpose1/1
  前轮侧向向量/1(eg_long) -> [e_g_lat_nose], Matrix Multiply/2
  Hermitian Transpose1/1 -> Matrix Multiply/1
  [V_left_g] -> Hermitian Transpose2/1
  [V_right_g] -> Hermitian Transpose3/1
  主轮侧向方向向量/1(eg_long) -> Matrix Multiply2/2, Matrix Multiply1/2, [e_g_lat_main]
  Hermitian Transpose3/1 -> Matrix Multiply1/1
  Hermitian Transpose2/1 -> Matrix Multiply2/1
  Matrix Multiply/1 -> V_lat_nose/1, [V_lat_nose]
  Matrix Multiply2/1 -> V_lat_left/1, [V_lat_left]
  Matrix Multiply1/1 -> V_lat_right/1, [V_lat_right]
  Cos/1 -> Mux/3
  Sin/1 -> Gain/1
  Gain/1 -> Mux/1
  delt-s(H)/1 -> Sin/1, Cos/1
  [theta_eular] -> MATLAB Function1/2(theta)
  [psi_eular] -> MATLAB Function1/3(psi)
  Reshape/1 -> 前轮侧向向量/2(eb_long)
  Reshape1/1 -> 主轮侧向方向向量/2(eb_long)

== system planmodel2023/6DOF-MODEL/动力学/起落架模型/侧向力/Subsystem1 ==
  In1 : Inport
  Constant5 : Constant  Value=0
  Switch : Switch  Criteria=u2 > Threshold  SaturateOnIntegerOverflow=off  InputSameDT=off
  F_lat_left : Outport
  wires:
  In1/1 -> Switch/1
  Constant5/1 -> Switch/3
  Switch/1 -> F_lat_left/1
  [contact_left] -> Switch/2

== system planmodel2023/6DOF-MODEL/动力学/起落架模型/侧向力/Subsystem2 ==
  In1 : Inport
  Constant5 : Constant  Value=0
  Switch : Switch  Criteria=u2 > Threshold  SaturateOnIntegerOverflow=off  InputSameDT=off
  F_lat_nose : Outport
  wires:
  In1/1 -> Switch/1
  Constant5/1 -> Switch/3
  Switch/1 -> F_lat_nose/1
  [contact_nose] -> Switch/2

== system planmodel2023/6DOF-MODEL/动力学/起落架模型/侧向力/Subsystem3 ==
  In1 : Inport
  Constant5 : Constant  Value=0
  Switch : Switch  Criteria=u2 > Threshold  SaturateOnIntegerOverflow=off  InputSameDT=off
  F_lat_right : Outport
  wires:
  [contact_right] -> Switch/2
  Switch/1 -> F_lat_right/1
  Constant5/1 -> Switch/3
  In1/1 -> Switch/1

== system planmodel2023/6DOF-MODEL/动力学/起落架模型/法向支反力/Subsystem ==
  In1 : Inport
  Constant5 : Constant  Value=0
  Switch : Switch  Criteria=u2 > Threshold  SaturateOnIntegerOverflow=off  InputSameDT=off
  N_nose : Outport
  wires:
  In1/1 -> Switch/1
  Constant5/1 -> Switch/3
  Switch/1 -> N_nose/1
  [contact_nose] -> Switch/2

== system planmodel2023/6DOF-MODEL/动力学/起落架模型/法向支反力/Subsystem1 ==
  In1 : Inport
  Constant5 : Constant  Value=0
  Switch : Switch  Criteria=u2 > Threshold  SaturateOnIntegerOverflow=off  InputSameDT=off
  N_left : Outport
  wires:
  [contact_left] -> Switch/2
  Switch/1 -> N_left/1
  Constant5/1 -> Switch/3
  In1/1 -> Switch/1

== system planmodel2023/6DOF-MODEL/动力学/起落架模型/法向支反力/Subsystem2 ==
  In1 : Inport
  Constant5 : Constant  Value=0
  Switch : Switch  Criteria=u2 > Threshold  SaturateOnIntegerOverflow=off  InputSameDT=off
  N_right : Outport
  wires:
  In1/1 -> Switch/1
  Constant5/1 -> Switch/3
  Switch/1 -> N_right/1
  [contact_right] -> Switch/2

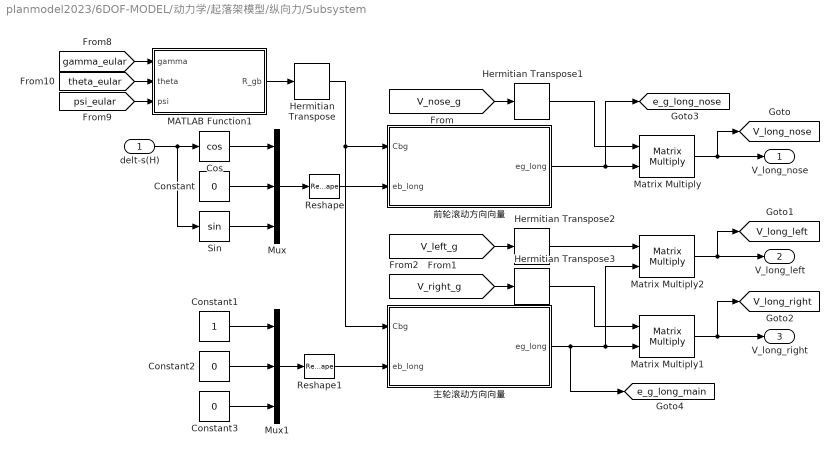
== system planmodel2023/6DOF-MODEL/动力学/起落架模型/纵向力/Subsystem ==
  delt-s(H) : Inport
  Constant : Constant  Value=0
  Constant1 : Constant
  Constant2 : Constant  Value=0
  Constant3 : Constant  Value=0
  Cos : Trigonometry  Operator=cos
  Hermitian Transpose{,1..3} (4 alike) : matrix_library/Hermitian Transpose
  MATLAB Function1 : MATLAB Function  TreatAsAtomicUnit=on
  Matrix Multiply : Product  Multiplication=Matrix(*)
  Matrix Multiply1 : Product  Multiplication=Matrix(*)
  Matrix Multiply2 : Product  Multiplication=Matrix(*)
  Mux : Mux  Inputs=3
  Mux1 : Mux  Inputs=3
  Reshape : Reshape  OutputDimensionality=Column vector (2-D)
  Reshape1 : Reshape  OutputDimensionality=Column vector (2-D)
  Sin : Trigonometry
  主轮滚动方向向量 : MATLAB Function  TreatAsAtomicUnit=on
  前轮滚动方向向量 : MATLAB Function  TreatAsAtomicUnit=on
  V_long_nose : Outport
  V_long_left : Outport  Port=2
  V_long_right : Outport  Port=3
  tag scope: V_long_left=global, V_long_nose=global, V_long_right=global, e_g_long_main=global, e_g_long_nose=global
  wires:
  MATLAB Function1/1(R_gb) -> Hermitian Transpose/1
  [gamma_eular] -> MATLAB Function1/1(gamma)
  Hermitian Transpose/1 -> 主轮滚动方向向量/1(Cbg), 前轮滚动方向向量/1(Cbg)
  delt-s(H)/1 -> Cos/1, Sin/1
  Cos/1 -> Mux/1
  Constant/1 -> Mux/2
  Sin/1 -> Mux/3
  Mux/1 -> Reshape/1
  Constant1/1 -> Mux1/1
  Constant2/1 -> Mux1/2
  Constant3/1 -> Mux1/3
  Mux1/1 -> Reshape1/1
  [V_nose_g] -> Hermitian Transpose1/1
  前轮滚动方向向量/1(eg_long) -> [e_g_long_nose], Matrix Multiply/2
  Hermitian Transpose1/1 -> Matrix Multiply/1
  [V_left_g] -> Hermitian Transpose2/1
  [V_right_g] -> Hermitian Transpose3/1
  主轮滚动方向向量/1(eg_long) -> Matrix Multiply1/2, Matrix Multiply2/2, [e_g_long_main]
  Hermitian Transpose3/1 -> Matrix Multiply1/1
  Hermitian Transpose2/1 -> Matrix Multiply2/1
  Matrix Multiply/1 -> V_long_nose/1, [V_long_nose]
  Matrix Multiply2/1 -> V_long_left/1, [V_long_left]
  Matrix Multiply1/1 -> V_long_right/1, [V_long_right]
  [theta_eular] -> MATLAB Function1/2(theta)
  [psi_eular] -> MATLAB Function1/3(psi)
  Reshape/1 -> 前轮滚动方向向量/2(eb_long)
  Reshape1/1 -> 主轮滚动方向向量/2(eb_long)

== system planmodel2023/6DOF-MODEL/动力学/起落架模型/纵向力/Subsystem1 ==
  V_long_nose : Inport
  V_long_left : Inport  Port=2
  V_long_right : Inport  Port=3
  u_brake : Inport  Port=4
  Add : Sum
  Add1 : Sum
  Add2 : Sum
  Constant : Constant  Value=v_eps
  Divide : Product  Inputs=*/
  Divide1 : Product  Inputs=*/
  Divide2 : Product  Inputs=*/
  Subsystem : Subsystem
  Subsystem1 : Subsystem
  Subsystem2 : Subsystem
  Subsystem3 : Subsystem
  Subsystem4 : Subsystem
  Tanh : Trigonometry  Operator=tanh
  Tanh1 : Trigonometry  Operator=tanh
  Tanh2 : Trigonometry  Operator=tanh
  F_long_nose : Outport
  F_long_left : Outport  Port=2
  F_long_right : Outport  Port=3
  wires:
  Divide1/1 -> Tanh1/1
  V_long_right/1 -> Divide2/1
  Divide2/1 -> Tanh2/1
  Constant/1 -> Divide1/2, Divide/2, Divide2/2
  Divide/1 -> Tanh/1
  V_long_left/1 -> Divide1/1
  V_long_nose/1 -> Divide/1
  u_brake/1 -> Subsystem/4(u_brake)
  Subsystem1/1(F_roll_nose) -> Add/1
  Subsystem1/2(F_roll_left) -> Add1/1
  Subsystem1/3(F_roll_right) -> Add2/1
  Subsystem/1(F_brake_nose) -> Add/2
  Subsystem/2(F_brake_left) -> Add1/2
  Subsystem/3(F_brake_right) -> Add2/2
  Tanh/1 -> Subsystem1/1(sig_nose), Subsystem/1(sig_nose)
  Tanh1/1 -> Subsystem1/2(sig_left), Subsystem/2(sig_left)
  Tanh2/1 -> Subsystem1/3(sig_right), Subsystem/3(sig_right)
  Add/1 -> Subsystem2/1(In1)
  Add1/1 -> Subsystem3/1(In1)
  Add2/1 -> Subsystem4/1(In1)
  Subsystem2/1(F_long_nose) -> F_long_nose/1
  Subsystem3/1(F_long_left) -> F_long_left/1
  Subsystem4/1(F_long_right) -> F_long_right/1

== system planmodel2023/control/俯仰通道控制器/俯仰通道/伪攻角回路/Subsystem ==
  Add : Sum
  Constant : Constant  Value=CLa
  Constant1 : Constant  Value=S_ref
  Constant2 : Constant  Value=m
  Constant3 : Constant  Value=D0
  Divide : Product  Inputs=*/
  Product : Product  Inputs=3
  Product1 : Product
  a34 : Outport
  wires:
  Constant/1 -> Product/1
  Constant1/1 -> Product/2
  [qc] -> Product/3
  Divide/1 -> a34/1
  [Va_safe] -> Product1/2
  Constant2/1 -> Product1/1
  Product1/1 -> Divide/2
  Constant3/1 -> Add/1
  Product/1 -> Add/2
  Add/1 -> Divide/1

== system planmodel2023/control/航向通道控制器/偏航通道/伪攻角回路/Subsystem ==
  Constant : Constant  Value=CSb
  Constant1 : Constant  Value=S_ref
  Constant2 : Constant  Value=m
  Constant3 : Constant  Value=D0
  Divide : Product  Inputs=*/
  Product : Product  Inputs=3
  Product1 : Product
  Subtract : Sum  Inputs=+-
  b : Outport
  wires:
  Constant/1 -> Product/1
  Constant1/1 -> Product/2
  [qc] -> Product/3
  Divide/1 -> b/1
  [Va_safe] -> Product1/2
  Constant2/1 -> Product1/1
  Product1/1 -> Divide/2
  Constant3/1 -> Subtract/1
  Product/1 -> Subtract/2
  Subtract/1 -> Divide/1

== system planmodel2023/control/航向通道控制器1/偏航通道/伪攻角回路/Subsystem ==
  Constant : Constant  Value=CSb
  Constant1 : Constant  Value=S_ref
  Constant2 : Constant  Value=m
  Constant3 : Constant  Value=D0
  Divide : Product  Inputs=*/
  Product : Product  Inputs=3
  Product1 : Product
  Subtract : Sum  Inputs=+-
  b : Outport
  wires:
  Constant/1 -> Product/1
  Constant1/1 -> Product/2
  [qc] -> Product/3
  Divide/1 -> b/1
  [Va_safe] -> Product1/2
  Constant2/1 -> Product1/1
  Product1/1 -> Divide/2
  Constant3/1 -> Subtract/1
  Product/1 -> Subtract/2
  Subtract/1 -> Divide/1

== system planmodel2023/6DOF-MODEL/动力学/起落架模型/纵向力/Subsystem1/Subsystem ==
  sig_nose : Inport
  sig_left : Inport  Port=2
  sig_right : Inport  Port=3
  u_brake : Inport  Port=4
  Constant2 : Constant  Value=mu_brake
  Demux1 : Demux  Outputs=3
  Gain3 : Gain  Gain=-1
  Product3 : Product  Inputs=4
  Product4 : Product  Inputs=4
  Product5 : Product  Inputs=4
  F_brake_nose : Outport
  F_brake_left : Outport  Port=2
  F_brake_right : Outport  Port=3
  wires:
  [N_nose] -> Product3/1
  Demux1/2 -> Product4/4
  [N_left] -> Product4/1
  Gain3/1 -> Product3/3, Product4/3, Product5/3
  [N_right] -> Product5/1
  Demux1/3 -> Product5/4
  u_brake/1 -> Gain3/1
  Constant2/1 -> Demux1/1
  Demux1/1 -> Product3/4
  sig_right/1 -> Product5/2
  Product3/1 -> F_brake_nose/1
  Product5/1 -> F_brake_right/1
  Product4/1 -> F_brake_left/1
  sig_nose/1 -> Product3/2
  sig_left/1 -> Product4/2

== system planmodel2023/6DOF-MODEL/动力学/起落架模型/纵向力/Subsystem1/Subsystem1 ==
  sig_nose : Inport
  sig_left : Inport  Port=2
  sig_right : Inport  Port=3
  Constant1 : Constant  Value=c_roll
  Demux : Demux  Outputs=3
  Gain : Gain  Gain=-1
  Gain1 : Gain  Gain=-1
  Gain2 : Gain  Gain=-1
  Product : Product  Inputs=3
  Product1 : Product  Inputs=3
  Product2 : Product  Inputs=3
  F_roll_nose : Outport
  F_roll_left : Outport  Port=2
  F_roll_right : Outport  Port=3
  wires:
  sig_left/1 -> Product1/3
  Demux/2 -> Product1/2
  Gain1/1 -> F_roll_left/1
  Constant1/1 -> Demux/1
  [N_nose] -> Product/1
  [N_left] -> Product1/1
  Product1/1 -> Gain1/1
  Demux/1 -> Product/2
  [N_right] -> Product2/1
  Demux/3 -> Product2/2
  Gain/1 -> F_roll_nose/1
  Product/1 -> Gain/1
  Product2/1 -> Gain2/1
  sig_right/1 -> Product2/3
  Gain2/1 -> F_roll_right/1
  sig_nose/1 -> Product/3

== system planmodel2023/6DOF-MODEL/动力学/起落架模型/纵向力/Subsystem1/Subsystem2 ==
  In1 : Inport
  Constant5 : Constant  Value=0
  Switch : Switch  Criteria=u2 > Threshold  SaturateOnIntegerOverflow=off  InputSameDT=off
  F_long_nose : Outport
  wires:
  In1/1 -> Switch/1
  Constant5/1 -> Switch/3
  Switch/1 -> F_long_nose/1
  [contact_nose] -> Switch/2

== system planmodel2023/6DOF-MODEL/动力学/起落架模型/纵向力/Subsystem1/Subsystem3 ==
  In1 : Inport
  Constant5 : Constant  Value=0
  Switch : Switch  Criteria=u2 > Threshold  SaturateOnIntegerOverflow=off  InputSameDT=off
  F_long_left : Outport
  wires:
  In1/1 -> Switch/1
  Constant5/1 -> Switch/3
  Switch/1 -> F_long_left/1
  [contact_left] -> Switch/2

== system planmodel2023/6DOF-MODEL/动力学/起落架模型/纵向力/Subsystem1/Subsystem4 ==
  In1 : Inport
  Constant5 : Constant  Value=0
  Switch : Switch  Criteria=u2 > Threshold  SaturateOnIntegerOverflow=off  InputSameDT=off
  F_long_right : Outport
  wires:
  [contact_right] -> Switch/2
  Switch/1 -> F_long_right/1
  Constant5/1 -> Switch/3
  In1/1 -> Switch/1

== matlab function planmodel2023/6DOF-MODEL/动力学/起落架模型/侧向力/Subsystem/MATLAB Function1 ==
  data: gamma input; R_gb output; theta input; psi input
function R_gb = ground2body(gamma, theta, psi)
    T1=[cos(psi), 0 ,-sin(psi);...
          0     , 1 ,    0   ;...
        sin(psi), 0 ,cos(psi);];%绕y偏航
    T2=[cos(theta),sin(theta),0;...
        -sin(theta),cos(theta),0;...
          0        , 0 ,       1;];%绕z俯仰角
    T3=[1,0,0;...
        0,cos(gamma),sin(gamma);...
        0,-sin(gamma),cos(gamma);];%绕x滚转角

   R_gb=T3*T2*T1;

== matlab function planmodel2023/6DOF-MODEL/动力学/起落架模型/侧向力/Subsystem/主轮侧向方向向量 ==
  data: Cbg input; eg_long output; eb_long input
function eg_long= project_long(Cbg,eb_long)


e_y=[0;1;0];
P_g=eye(3)-e_y*e_y';

eg_long=P_g*Cbg*eb_long;
eg_long=eg_long/norm(eg_long);

== matlab function planmodel2023/6DOF-MODEL/动力学/起落架模型/侧向力/Subsystem/前轮侧向向量 ==
  data: Cbg input; eg_long output; eb_long input
function eg_long= project_long(Cbg,eb_long)


e_y=[0;1;0];
P_g=eye(3)-e_y*e_y';

eg_long=P_g*Cbg*eb_long;
eg_long=eg_long/norm(eg_long);

== matlab function planmodel2023/6DOF-MODEL/动力学/起落架模型/MATLAB Function1 ==
  data: gamma input; R_gb output; theta input; psi input
function R_gb = ground2body(gamma, theta, psi)
    T1=[cos(psi), 0 ,-sin(psi);...
          0     , 1 ,    0   ;...
        sin(psi), 0 ,cos(psi);];%绕y偏航
    T2=[cos(theta),sin(theta),0;...
        -sin(theta),cos(theta),0;...
          0        , 0 ,       1;];%绕z俯仰角
    T3=[1,0,0;...
        0,cos(gamma),sin(gamma);...
        0,-sin(gamma),cos(gamma);];%绕x滚转角

   R_gb=T3*T2*T1;

== matlab function planmodel2023/6DOF-MODEL/动力学/起落架模型/MATLAB Function2 ==
  data: gamma input; R_gb output; theta input; psi input
function R_gb = ground2body(gamma, theta, psi)
    T1=[cos(psi), 0 ,-sin(psi);...
          0     , 1 ,    0   ;...
        sin(psi), 0 ,cos(psi);];%绕y偏航
    T2=[cos(theta),sin(theta),0;...
        -sin(theta),cos(theta),0;...
          0        , 0 ,       1;];%绕z俯仰角
    T3=[1,0,0;...
        0,cos(gamma),sin(gamma);...
        0,-sin(gamma),cos(gamma);];%绕x滚转角

   R_gb=T3*T2*T1;

== matlab function planmodel2023/6DOF-MODEL/动力学/起落架模型/三轮在地系下的力/摩擦圆限幅/前轮摩擦圆限幅 ==
  data: N input; F_long_out output; F_long input; F_lat input; F_lat_out output
function [F_long_out,F_lat_out]=Dround_saturation_nose(N,F_long,F_lat)
mu=0.65;
F_ALL=sqrt((F_long)^2+(F_lat)^2);
if(F_ALL<=mu*N)
    F_long_out=F_long;
    F_lat_out=F_lat;
else
    s=mu*N/F_ALL;
    F_long_out=s*F_long;
    F_lat_out=s*F_lat;
end

== matlab function planmodel2023/6DOF-MODEL/动力学/起落架模型/三轮在地系下的力/摩擦圆限幅/主轮摩擦圆限幅左 ==
  data: N input; F_long_out output; F_long input; F_lat input; F_lat_out output
function [F_long_out,F_lat_out]=Dround_saturation_main(N,F_long,F_lat)
mu=0.7;
F_ALL=sqrt((F_long)^2+(F_lat)^2);
if(F_ALL<=mu*N)
    F_long_out=F_long;
    F_lat_out=F_lat;
else
    s=mu*N/F_ALL;
    F_long_out=s*F_long;
    F_lat_out=s*F_lat;
end

== matlab function planmodel2023/6DOF-MODEL/动力学/起落架模型/三轮在地系下的力/摩擦圆限幅/主轮摩擦圆限幅右 ==
  data: N input; F_long_out output; F_long input; F_lat input; F_lat_out output
function [F_long_out,F_lat_out]=Dround_saturation_main(N,F_long,F_lat)
mu=0.7;
F_ALL=sqrt((F_long)^2+(F_lat)^2);
if(F_ALL<=mu*N)
    F_long_out=F_long;
    F_lat_out=F_lat;
else
    s=mu*N/F_ALL;
    F_long_out=s*F_long;
    F_lat_out=s*F_lat;
end

== matlab function planmodel2023/control/俯仰通道控制器/MATLAB Function ==
  settings: updateMethod=DISCRETE
  data: Vx input; theta_cmd output; no_contact input; t input; theta_actual input
function theta_cmd = fcn(Vx, no_contact, t, theta_actual)
% 起飞抬前轮俯仰角指令生成
% Vx:           机体系前向速度 (m/s)
% no_contact:   无轮接地信号, 1=空中, 0=地面
% t:            仿真时间 (s), 接 Digital Clock
% theta_actual: 飞机当前的实际俯仰角 (rad), 用于离地无缝切换

persistent t_rotation
persistent theta_takeoff_hold

if isempty(t_rotation)
    t_rotation = inf;
end
if isempty(theta_takeoff_hold)
    theta_takeoff_hold = 0;
end

%% --- 参数配置
VR = 65;                      % m/s, 抬轮速度 
theta_target = 4 * pi/180;   % rad,
rotation_rate = 0.5 * pi/180;   % rad/s

%% --- 状态机控制逻辑 ---
if no_contact > 0.5
    % 【空中阶段】
    % 刚离地瞬间，记录下离地时的实际姿态，防止指令断崖式下掉
    if theta_takeoff_hold == 0
        theta_takeoff_hold = theta_actual; 
    end

    theta_cmd = theta_takeoff_hold; 
    
    % 重置滑跑计时器
    t_rotation = inf;

elseif Vx >= VR
    % 【抬轮阶段】
    if isinf(t_rotation)
        t_rotation = t;       % 记录开始抬轮的绝对时间
    end
    
    % 按照设定的速率（3°/s）线性增加俯仰角指令
    theta_cmd = rotation_rate * (t - t_rotation);
    
    % 达到目标角度（10°）后进行限幅切顶
    if theta_cmd > theta_target
        theta_cmd = theta_target;
    end
    
    % 尚未离地，清空离地保持值
    theta_takeoff_hold = 0;

else
    % 【地面加速滑跑阶段】
    % 保持前轮三点接地姿态（通常为 0° 或略微带一点下俯角压前轮，视安装角而定）
    theta_cmd = -10*pi/180; 
    t_rotation = inf;
    theta_takeoff_hold = 0;
end% 在你的状态机逻辑中添加：

end

== matlab function planmodel2023/6DOF-MODEL/动力学/体系旋转角速度/MATLAB Function ==
  data: alpha input; R_wind_b output; beta input
 function R_wind_b = wind2body(alpha, beta)
T1 = [cos(beta), 0, -sin(beta);
       0, 1, 0;
       sin(beta), 0, cos(beta)];
T2 = [cos(alpha), sin(alpha), 0;
       -sin(alpha), cos(alpha), 0;
       0, 0, 1];
R_wind_b = T2*T1;

== matlab function planmodel2023/6DOF-MODEL/动力学/Subsystem3/MATLAB Function1 ==
  data: gamma input; R_gb output; theta input; psi input
function R_gb = ground2body(gamma, theta, psi)
    T1=[cos(psi), 0 ,-sin(psi);...
          0     , 1 ,    0   ;...
        sin(psi), 0 ,cos(psi);];%绕y偏航
    T2=[cos(theta),sin(theta),0;...
        -sin(theta),cos(theta),0;...
          0        , 0 ,       1;];%绕z俯仰角
    T3=[1,0,0;...
        0,cos(gamma),sin(gamma);...
        0,-sin(gamma),cos(gamma);];%绕x滚转角

   R_gb=T3*T2*T1;

== matlab function planmodel2023/6DOF-MODEL/动力学/起落架模型/起落架三轮质心在地系下位置/MATLAB Function1 ==
  data: gamma input; R_gb output; theta input; psi input
function R_gb = ground2body(gamma, theta, psi)
    T1=[cos(psi), 0 ,-sin(psi);...
          0     , 1 ,    0   ;...
        sin(psi), 0 ,cos(psi);];%绕y偏航
    T2=[cos(theta),sin(theta),0;...
        -sin(theta),cos(theta),0;...
          0        , 0 ,       1;];%绕z俯仰角
    T3=[1,0,0;...
        0,cos(gamma),sin(gamma);...
        0,-sin(gamma),cos(gamma);];%绕x滚转角

   R_gb=T3*T2*T1;

== matlab function planmodel2023/6DOF-MODEL/动力学/height/MATLAB Function2 ==
  data: gamma input; R_gb output; theta input; psi input
function R_gb = ground2body(gamma, theta, psi)
    T1=[cos(psi), 0 ,-sin(psi);...
          0     , 1 ,    0   ;...
        sin(psi), 0 ,cos(psi);];%绕y偏航
    T2=[cos(theta),sin(theta),0;...
        -sin(theta),cos(theta),0;...
          0        , 0 ,       1;];%绕z俯仰角
    T3=[1,0,0;...
        0,cos(gamma),sin(gamma);...
        0,-sin(gamma),cos(gamma);];%绕x滚转角

   R_gb=T3*T2*T1;
